simulink model "Berghuis_Cook"  (R2017a)
settings: Solver=FixedStepAuto  StartTime=0.0  StopTime=10  FixedStep=dt  RelTol=1e-3
values from neighbouring files (symbols this model uses):
  alpha12 = 20    [Berghuis_Cook_init.m]
  c = 2*zeta*sqrt(m*k)    [Berghuis_Cook_init.m]
  dt = 1e-4    (= 0.0001)    [Berghuis_Cook_init.m]
  k = m * wn^2    (= 4934802.20054)    [Berghuis_Cook_init.m]
  m = 0.125    [Berghuis_Cook_init.m]
  P = Pr*10^(db/20)    (= 0.0632455532034)    [Berghuis_Cook_init.m]
  sinFreq = sinHz.*2*pi    [Berghuis_Cook_init.m]
settings Model: Creator=212454356  LastModifiedBy=212454356
settings DebuggingCC: UniqueDataStoreMsg=error

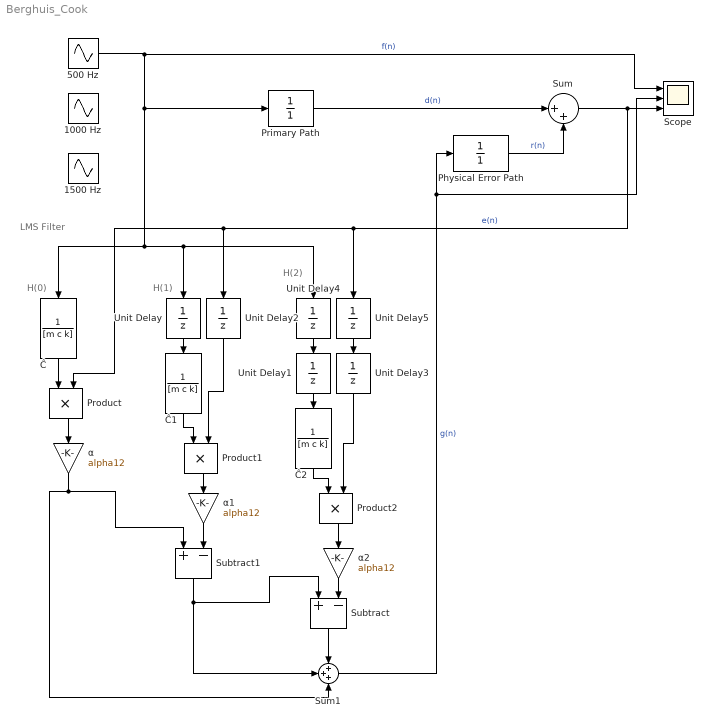
== system Berghuis_Cook ==
  note: H(2)
  note: H(1)
  note: H(0)
  note: LMS Filter
  1000 Hz : Sin  Amplitude=P  Frequency=sinFreq(2)  SampleTime=0
  1500 Hz : Sin  Amplitude=P  Frequency=sinFreq(3)  SampleTime=0
  500 Hz : Sin  Amplitude=P  Frequency=sinFreq(1)  SampleTime=0
  Physical Error Path : TransferFcn  Denominator=[1]
  Primary Path : TransferFcn  Denominator=[1]
  Product : Product
  Product1 : Product
  Product2 : Product
  Scope : Scope  NumInputPorts=3
  Subtract : Sum  Inputs=+-
  Subtract1 : Sum  Inputs=+-
  Sum : Sum  Inputs=|++
  Sum1 : Sum  Inputs=3
  Unit Delay{,1..5} (6 alike) : UnitDelay  SampleTime=dt
  Ĉ : TransferFcn  Denominator=[m c k]
  Ĉ1 : TransferFcn  Denominator=[m c k]
  Ĉ2 : TransferFcn  Denominator=[m c k]
  α : Gain  Gain=alpha12
  α1 : Gain  Gain=alpha12
  α2 : Gain  Gain=alpha12
  wires:
  Primary Path/1 -> Sum/1  "d(n)"
  Physical Error Path/1 -> Sum/2  "r(n)"
  500 Hz/1 -> Scope/1, Primary Path/1, Unit Delay/1, Unit Delay4/1, Ĉ/1  "f(n)"
  Sum/1 -> Product/2, Unit Delay2/1, Unit Delay5/1, Scope/3  "e(n)"
  Sum1/1 -> Scope/2, Physical Error Path/1  "g(n)"
  α/1 -> Sum1/3, Subtract1/1
  Unit Delay/1 -> Ĉ1/1
  α1/1 -> Subtract1/2
  Unit Delay2/1 -> Product1/2
  Unit Delay1/1 -> Ĉ2/1
  Unit Delay4/1 -> Unit Delay1/1
  Subtract1/1 -> Subtract/1, Sum1/2
  Subtract/1 -> Sum1/1
  α2/1 -> Subtract/2
  Unit Delay5/1 -> Unit Delay3/1
  Unit Delay3/1 -> Product2/2
  Ĉ/1 -> Product/1
  Product/1 -> α/1
  Ĉ1/1 -> Product1/1
  Product1/1 -> α1/1
  Ĉ2/1 -> Product2/1
  Product2/1 -> α2/1
